simulink model "class_2_simulink1"  (R2023b)
settings: Solver=VariableStepAuto  StartTime=0.0  StopTime=10.0  RelTol=1e-3
undefined symbols (not defined in the file or in its folder): denp, nump
libraries: cstblocks x4
settings Model: Creator=klysm  LastModifiedBy=klysm

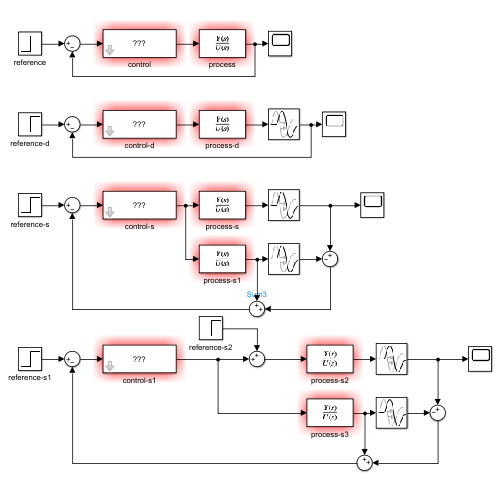
[thumbnail: Simulink's stored preview of the top-level diagram]
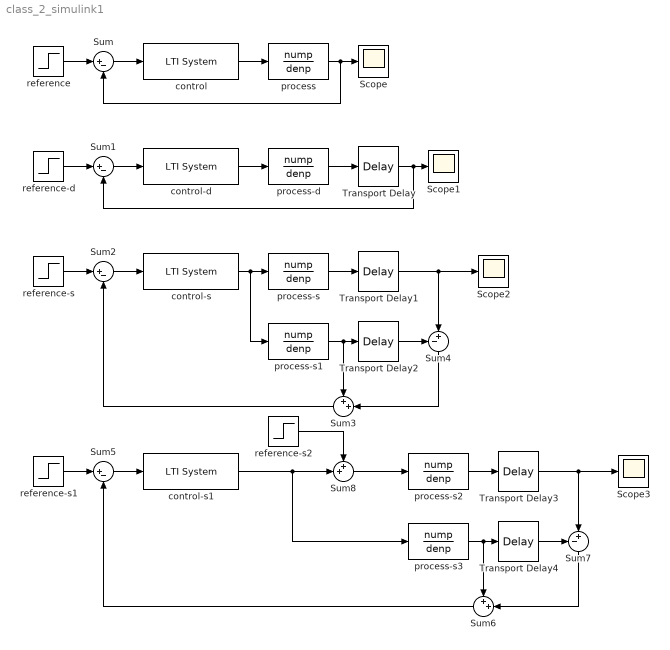
== system class_2_simulink1 ==
  Scope{,1..3} (4 alike) : Scope
  Sum{,1..2,5} (4 alike) : Sum  Inputs=|+-
  Sum3 : Sum  Inputs=++|
  Sum4 : Sum  Inputs=-+|
  Sum6 : Sum  Inputs=++|
  Sum7 : Sum  Inputs=-+|
  Sum8 : Sum  Inputs=++|
  Transport Delay{,1..4} (5 alike) : TransportDelay
  control : cstblocks/LTI System  sys=C  IC=[]  PadeOrder=0
  control-d : cstblocks/LTI System  sys=C  IC=[]  PadeOrder=0
  control-s : cstblocks/LTI System  sys=C  IC=[]  PadeOrder=0
  control-s1 : cstblocks/LTI System  sys=C  IC=[]  PadeOrder=0
  process : TransferFcn  Numerator=nump  Denominator=denp
  process-d : TransferFcn  Numerator=nump  Denominator=denp
  process-s{,1..3} (4 alike) : TransferFcn  Numerator=nump  Denominator=denp
  reference : Step  SampleTime=0
  reference-d : Step  SampleTime=0
  reference-s : Step  SampleTime=0
  reference-s1 : Step  SampleTime=0
  reference-s2 : Step  SampleTime=0
  wires:
  reference/1 -> Sum/1
  control/1 -> process/1
  Sum/1 -> control/1
  process/1 -> Sum/2, Scope/1
  process-d/1 -> Transport Delay/1
  Sum1/1 -> control-d/1
  reference-d/1 -> Sum1/1
  control-d/1 -> process-d/1
  Transport Delay/1 -> Sum1/2, Scope1/1
  control-s/1 -> process-s1/1, process-s/1
  Sum2/1 -> control-s/1
  process-s/1 -> Transport Delay1/1
  Transport Delay1/1 -> Scope2/1, Sum4/2
  reference-s/1 -> Sum2/1
  process-s1/1 -> Sum3/1, Transport Delay2/1
  Sum4/1 -> Sum3/2
  Transport Delay2/1 -> Sum4/1
  Sum3/1 -> Sum2/2
  Sum6/1 -> Sum5/2
  Sum7/1 -> Sum6/2
  Sum5/1 -> control-s1/1
  process-s2/1 -> Transport Delay3/1
  control-s1/1 -> Sum8/2, process-s3/1
  Transport Delay4/1 -> Sum7/1
  reference-s1/1 -> Sum5/1
  process-s3/1 -> Sum6/1, Transport Delay4/1
  Transport Delay3/1 -> Scope3/1, Sum7/2
  Sum8/1 -> process-s2/1
  reference-s2/1 -> Sum8/1
